simulink model "SpeedControl"  (R2021a)
settings: Solver=VariableStepAuto  StartTime=0.0  StopTime=10  RelTol=1e-3
undefined symbols (not defined in the file): sigbuilder_block
libraries: spsIGBTDiodeLib x6, spsThreePhaseSineGeneratorLib x1, spsDCVoltageSourceLib x1, simulink x1, spsAsynchronousMachineSIUnitsLib x1, spsThreePhaseVIMeasurementLib x1, spspowerguiLib x1
settings Model: Creator=DELL  LastModifiedBy=DELL

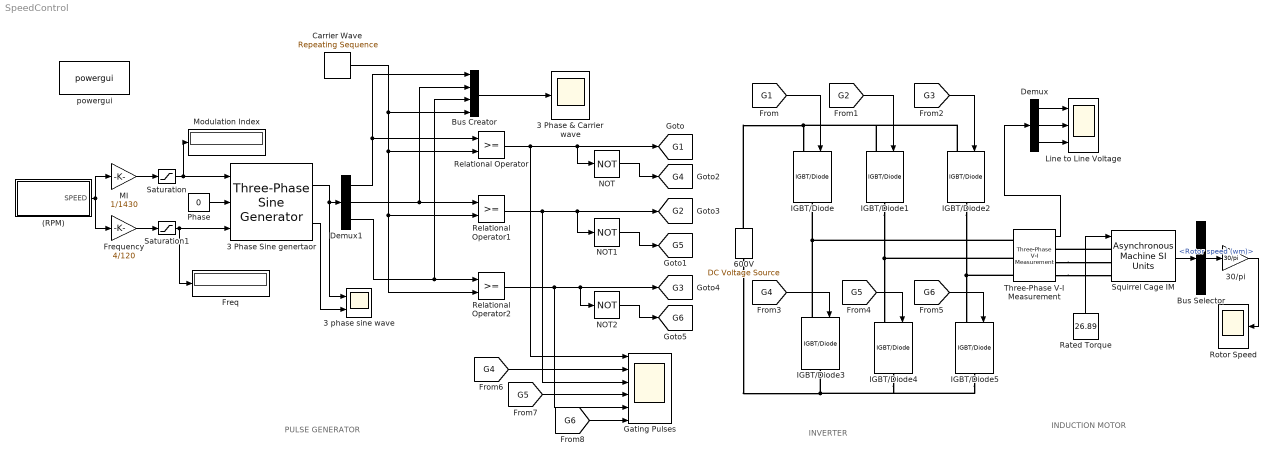
== system SpeedControl ==
  note: INDUCTION MOTOR
  note: PULSE GENERATOR
  note: INVERTER
  (RPM) : Subsystem  Tag=STV Subsys  LoadFcn=sigbuilder_block('load');  StartFcn=sigbuilder_block('start');  StopFcn=sigbuilder_block('stop');  ClipboardFcn=sigbuilder_block('clipboard');  mask(Sigbuilder block){tuvar=[0:10]}
      mask help: Simulink:masks:SigbuilderBlock_MD
      mask init:
      | if ~strcmp(get_param(bdroot(gcbh),'SimulationStatus'),'stopped') tuvar = sigbuilder_block('maskInit'); end
      settings: CopyFcn=sigbuilder_block('copy');  DeleteFcn=sigbuilder_block('delete');  ModelCloseFcn=sigbuilder_block('modelClose');  PreSaveFcn=sigbuilder_block('preSave');  PauseFcn=sigbuilder_block('pause');  ContinueFcn=sigbuilder_block('continue');  NameChangeFcn=sigbuilder_block('namechange');  OpenFcn=sigbuilder_block('open',[406.2 141.6 550.8 400.2 ]);  CloseFcn=sigbuilder_block('close');
      mask Display: plot(0, 0, 100, 100,[2, 2, 32, 32, 2], [68, 8, 8, 68, 68],[32, 2], [38, 38], [32, 19, 2],[53, 60, 44], [32, 17, 17, 2],[16, 16, 31, 31]);txt = getActiveGroup(gcbh);text(2, 100, txt,'verticalAlignment', 'top');
  3 Phase & Carrier wave : Scope
  3 Phase Sine genertaor : spsThreePhaseSineGeneratorLib/Three-Phase Sine Generator  Ts=0
      settings: SourceProductBaseCode=PS
  3 phase sine wave : Scope  NumInputPorts=2
  30/pi : Gain  Gain=30/pi
  600V : spsDCVoltageSourceLib/DC Voltage Source  Amplitude=600  Measurements=None
  Bus Creator : BusCreator  Inputs=4
  Bus Selector : BusSelector  OutputSignals=Mechanical.Rotor speed (wm)
  Carrier Wave : simulink/Sources/Repeating Sequence  rep_seq_t=[0 0.25 0.5 0.75 1]/1000  rep_seq_y=[0 1 0 -1 0]
  Demux : Demux  Outputs=3
  Demux1 : Demux  Outputs=3
  Freq : Display
  Frequency : Gain  Gain=4/120
  Gating Pulses : Scope  NumInputPorts=6
  IGBT/Diode{,1..5} (6 alike) : spsIGBTDiodeLib/IGBT//Diode  Ron=1e-3  Rs=1e5  Cs=inf  Measurements=off
  Line to Line Voltage : Scope  NumInputPorts=3
  MI : Gain  Gain=1/1430
  Modulation Index : Display
  NOT : Logic  Operator=NOT  IconShape=distinctive  AllPortsSameDT=off  OutDataTypeStr=boolean
  NOT1 : Logic  Operator=NOT  IconShape=distinctive  AllPortsSameDT=off  OutDataTypeStr=boolean
  NOT2 : Logic  Operator=NOT  IconShape=distinctive  AllPortsSameDT=off  OutDataTypeStr=boolean
  Phase : Constant  Value=0
  Rated Torque : Constant  Value=26.89
  Relational Operator : RelationalOperator  OutDataTypeStr=boolean  RndMeth=Simplest
  Relational Operator1 : RelationalOperator  OutDataTypeStr=boolean  RndMeth=Simplest
  Relational Operator2 : RelationalOperator  OutDataTypeStr=boolean  RndMeth=Simplest
  Rotor Speed : Scope
  Saturation : Saturate  UpperLimit=1  LowerLimit=0.1
  Saturation1 : Saturate  UpperLimit=50  LowerLimit=2
  Squirrel Cage IM : spsAsynchronousMachineSIUnitsLib/Asynchronous Machine SI Units  RotorType=Squirrel-cage  PresetModel="15:  5.4 HP (4KW)   400 V  50Hz 1430 RPM"  MechanicalLoad=Torque Tm  ShowDetailedParameters=on  ReferenceFrame=Rotor  Units=SI  MeasurementBus=off  NominalParameters=[4000 400 50]  VoltageRatio=1  Stator=[1.405 0.005839]  Rotor=[1.395 0.005839]  Cage1=[0.4155 0.002066]  Cage2=[0.4168 0.0003495]  Lm=0.1722  Mechanical=[0.0131 0.002985 2]  PolePairs=2  InitialConditions=[0 0 0 0 0 0 0 0]  SimulateSaturation=off  Saturation=[14.03593122, 27.81365428, 53.79336849, 72.68890987, 97.98006896, 148.6815601, 215.7428561, 302.9841135, 428.7778367 ; 230, 322, 414, 460, 506, 552, 598, 644, 690]  LoadFlowParameters=1492000  TsPowergui=0  TsBlock=-1  IterativeModel=Trapezoidal non iterative  IterativeDiscreteModel=Trapezoidal non iterative  Pmec=1.492e+006
  Three-Phase V-I Measurement : spsThreePhaseVIMeasurementLib/Three-Phase V-I Measurement  VoltageMeasurement=phase-to-phase  SetLabelV=off  LabelV=phase-to-phase  Vpu=off  VpuLL=off  CurrentMeasurement=no  SetLabelI=off  LabelI=Iabc  Ipu=off  Pbase=100e6  Vbase=500e3  OutputType=Complex  PhasorSimulation=off  PSBequivalent=0
  powergui : spspowerguiLib/powergui  Priority=1  SimulationMode=Discrete  SampleTime=50e-6  frequency=60  Iterations=50  frequencyindice=0  Pbase=100e6  ErrMax=1e-4  UnitsV=kV  UnitsW=MW  buscounter=0  FunctionMessages=off  echomessages=off  EnableUseOfTLC=off  CurrentSourceSwitches=off  DisableSnubberDevices=off  DisableRonSwitches=off  DisableVfSwitches=off  DisplayEquations=off  AutomaticDiscreteSolvers=off  SolverType=Tustin/Backward Euler (TBE)  Interpol=off  ExternalGateDelay=off  methode=off  Ts=100  x0status=blocks  SPID=on  SwTol=0  HookPort=off  NonlinearTolerance=1e-4  nMaxIteration=100  ContinueOnMaxIteration=off  RestoreLinks=warning  ResistiveCurrentMeasurement=off  Frange=[0:2:500]  Ylog=off  Xlog=on  ShowGrid=off  save=off  variable=ZData  structure=0  ZoomFFT=off  StartTime=0.0  cycles=1  DisplayStyle=1  fundamental=60  FreqAxis=off  MaxFrequency=1000  frequencyindicesteady=1  RmsSteady=1  display=off
  tag scope: G1=global, G2=global, G3=global, G4=global, G5=global, G6=global
  wires:
  Demux1/2 -> Bus Creator/2, Relational Operator1/1
  Demux1/3 -> Bus Creator/3, Relational Operator2/1
  Carrier Wave/1 -> Bus Creator/4, Relational Operator/2, Relational Operator2/2, Relational Operator1/2
  Relational Operator/1 -> Gating Pulses/1, [G1], NOT/1
  Relational Operator2/1 -> Gating Pulses/5, [G3], NOT2/1
  Demux1/1 -> Bus Creator/1, Relational Operator/1
  [G4] -> IGBT/Diode3/1
  [G5] -> IGBT/Diode4/1
  [G6] -> IGBT/Diode5/1
  [G3] -> IGBT/Diode2/1
  [G2] -> IGBT/Diode1/1
  [G1] -> IGBT/Diode/1
  NOT1/1 -> [G5]
  Squirrel Cage IM/1 -> Bus Selector/1
  Bus Selector/1 -> 30/pi/1  "<Rotor speed (wm)>"
  Bus Creator/1 -> 3 Phase & Carrier wave/1
  NOT/1 -> [G4]
  Relational Operator1/1 -> Gating Pulses/3, NOT1/1, [G2]
  [G4] -> Gating Pulses/2
  [G5] -> Gating Pulses/4
  [G6] -> Gating Pulses/6
  30/pi/1 -> Rotor Speed/1
  Phase/1 -> 3 Phase Sine genertaor/2
  3 Phase Sine genertaor/1 -> 3 phase sine wave/1, Demux1/1
  Rated Torque/1 -> Squirrel Cage IM/1
  (RPM)/1(SPEED) -> MI/1, Frequency/1
  3 Phase Sine genertaor/2 -> 3 phase sine wave/2
  Demux/3 -> Line to Line Voltage/3
  Demux/2 -> Line to Line Voltage/2
  Three-Phase V-I Measurement/1 -> Demux/1
  Demux/1 -> Line to Line Voltage/1
  NOT2/1 -> [G6]
  Frequency/1 -> Saturation1/1
  Saturation1/1 -> Freq/1, 3 Phase Sine genertaor/3
  MI/1 -> Saturation/1
  Saturation/1 -> Modulation Index/1, 3 Phase Sine genertaor/1
  connections:
  IGBT/Diode1/LConn1 -- IGBT/Diode2/LConn1 -- IGBT/Diode/LConn1 -- 600V/RConn1
  IGBT/Diode3/LConn1 -- IGBT/Diode/RConn1 -- Three-Phase V-I Measurement/LConn1
  IGBT/Diode1/RConn1 -- Three-Phase V-I Measurement/LConn2 -- IGBT/Diode4/LConn1
  IGBT/Diode2/RConn1 -- Three-Phase V-I Measurement/LConn3 -- IGBT/Diode5/LConn1
  IGBT/Diode5/RConn1 -- IGBT/Diode4/RConn1 -- 600V/LConn1 -- IGBT/Diode3/RConn1
  Squirrel Cage IM/LConn1 -- Three-Phase V-I Measurement/RConn1
  Three-Phase V-I Measurement/RConn2 -- Squirrel Cage IM/LConn2
  Three-Phase V-I Measurement/RConn3 -- Squirrel Cage IM/LConn3

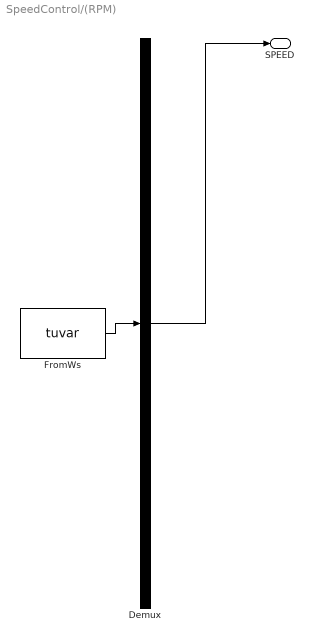
== system SpeedControl/(RPM) ==
  Demux : Demux  Tag=STV Demux  Outputs=1
      settings: DisplayOption=none
  FromWs : FromWorkspace  Tag=STV FromWs  VariableName=tuvar
      SigBuilderData=|
      | common.afterFinalStr = 'Extrapolate'
      | common.sampleTime = 0
      | dataSet.timeRange = [0 10]
      | dataSet.name = 'INPUT'
      | sbobj.Groups.Name = 'INPUT'
      | sbobj.Groups.Signals.Name = 'SPEED'
      | sbobj.Groups.Signals.XData = [0 4 4 6 6 10]
      | sbobj.Groups.Signals.YData = [1000 1000 1500 1500 500 500]
  SPEED : Outport  Tag=STV Outport
  wires:
  Demux/1 -> SPEED/1
  FromWs/1 -> Demux/1
